simulink model "lab_modulation_pm"  (R2022a)
settings: Solver=VariableStepAuto  StartTime=0.0  StopTime=10.0  RelTol=1e-3
libraries: dspfdesign x1, commanapbnd3 x1
settings Model: Creator=salgi  LastModifiedBy=salgi

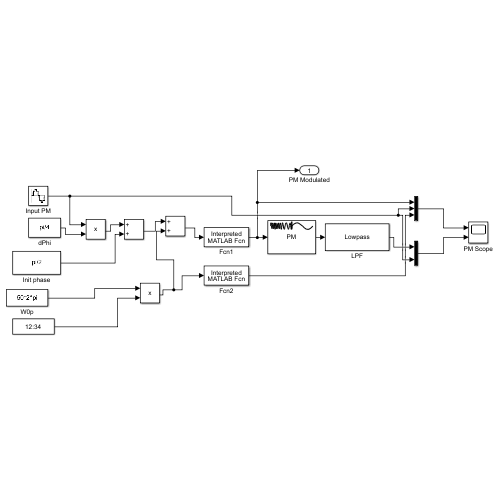
[thumbnail: Simulink's stored preview of the top-level diagram]
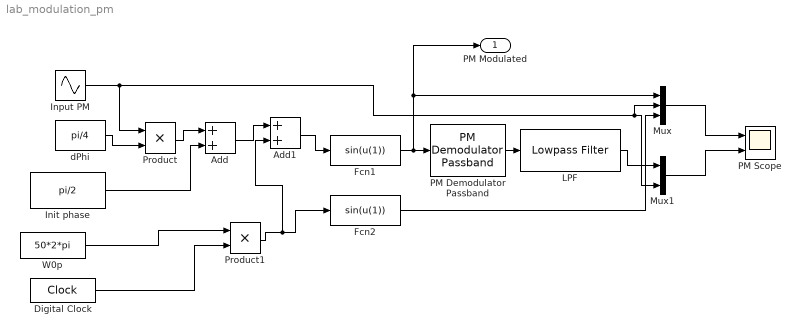
== system lab_modulation_pm ==
  Add : Sum
  Add1 : Sum
  Digital Clock : DigitalClock
  Fcn1 : MATLABFcn  MATLABFcn=sin(u(1))
  Fcn2 : MATLABFcn  MATLABFcn=sin(u(1))
  Init phase : Constant  Value=pi/2
  Input PM : Sin  Frequency=2*2*pi  SampleTime=0.0001
  LPF : dspfdesign/Lowpass Filter  FilterType=FIR  DesignForMinimumOrder=on  FilterOrder=50  PassbandFrequency=0.1  StopbandFrequency=100  PassbandRipple=0.1  StopbandAttenuation=80  InheritSampleRate=on  SampleRate=44100  SimulateUsing=Interpreted execution  roundingMode=Floor  coeffsDataTypeStr=fixdt(1,16)
  Mux : Mux  Inputs=3
  Mux1 : Mux  Inputs=2
  PM Demodulator Passband : commanapbnd3/PM Demodulator Passband  Fc=50  Ph=0  Kc=pi/4  Ho=100
      settings: SourceProductBaseCode=CM
  PM Scope : Scope  NumInputPorts=2
  Product : Product
  Product1 : Product
  W0p : Constant  Value=50*2*pi
  dPhi : Constant  Value=pi/4
  PM Modulated : Outport
  wires:
  Fcn2/1 -> Mux/3
  Init phase/1 -> Add/2
  PM Demodulator Passband/1 -> LPF/1
  dPhi/1 -> Product/2
  Fcn1/1 -> PM Modulated/1, Mux/1, PM Demodulator Passband/1
  Input PM/1 -> Product/1, Mux1/2, Mux/2
  Add/1 -> Add1/1
  Add1/1 -> Fcn1/1
  Product/1 -> Add/1
  Product1/1 -> Add1/2, Fcn2/1
  Mux/1 -> PM Scope/1
  W0p/1 -> Product1/1
  Digital Clock/1 -> Product1/2
  LPF/1 -> Mux1/1
  Mux1/1 -> PM Scope/2
